simulink library "sm_excv_scene_lib"  (R2023a)
settings: Solver=VariableStepAuto  StartTime=0.0  StopTime=10.0  RelTol=1e-3
undefined symbols (not defined in the file): B1, B2, B3, B4, B5, B6, B7, B8, Excv, L1, L2, L3, L4, L5, L6, L7, L8, L9, Road, S1, S2, Scene, Scene_Data, SceneData, X, Y, Z
libraries: sm_lib x65, sm_tracked_vehicle_lib x47, $bdroot x45, nesl_utility x10
(part 2 of 3)

== system sm_excv_scene_lib/Grid Surface Terrain 1 Track ==
  CF Track Terrain L : sm_tracked_vehicle_lib/CF Track Terrain Full  K_Road=Scene.Contact.Terrain.K  B_Road=Scene.Contact.Terrain.B  TW_Road=Scene.Contact.Terrain.TW  F_dyn_Road=Scene.Contact.Terrain.mud  F_stat_Road=Scene.Contact.Terrain.mus  CV_Road=Scene.Contact.Terrain.CV
      settings: LibrarySourceBlock=sm_chain_drive_lib/CF_Road_Full
  Grid Surface : sm_lib/Curves and Surfaces/Grid Surface  XGridVector=Scene.Terrain.xg  XGridVectorUnits=m  YGridVector=Scene.Terrain.yg  YGridVectorUnits=m  ZHeights=Scene.Terrain.z_heights_data  ZHeightsUnits=m  GraphicType=FromGeometry  GraphicVisPropType=SimpleVisualProperties  GraphicDiffuseColor=[0.8196 0.7255 0.5098]  GraphicOpacity=1.0  GraphicSpecularColor=[0.5 0.5 0.5 1.0]  GraphicAmbientColor=[0.15 0.15 0.15 1.0]  GraphicEmissiveColor=[0.0 0.0 0.0 1.0]  GraphicShininess=75
  Transform Terrain : sm_lib/Frames and Transforms/Rigid Transform  TranslationMethod=Cartesian  TranslationStandardOffset=0  TranslationStandardOffsetUnits=m  TranslationStandardAxis=+Z  TranslationCartesianOffset="[-45 -45+2.5  -2.75+0.2]"  TranslationCartesianOffsetUnits=m  TranslationROffset=0  TranslationROffsetUnits=m  TranslationZOffset=0  TranslationZOffsetUnits=m  TranslationThetaOffset=0  TranslationThetaOffsetUnits=deg  RotationMethod=None  RotationAngleUnits=deg  RotationStandardAxis=+Z  RotationAngle=0.0  RotationArbitraryAxis=[0 0 1]  FollAlignAxisA=+X  BaseAlignAxisA=+Y  FollAlignAxisB=+Y  BaseAlignAxisB=+Z  RotationSequenceAxes=FollowerAxes  RotationSequence=XYX  RotationSequenceAngles=[0 0 0]  RotationSequenceAnglesUnits=deg  RotationMatrix=[1 0 0; 0 1 0; 0 0 1]  Quaternion=[1 0 0 0]
  W : PMIOPort  Side=Right
  L : PMIOPort  Port=2  Side=Left
  connections:
  CF Track Terrain L/RConn1 -- L/RConn1
  Transform Terrain/RConn1 -- Grid Surface/LConn1
  Grid Surface/RConn1 -- CF Track Terrain L/LConn1
  Transform Terrain/LConn1 -- W/RConn1

== system sm_excv_scene_lib/Grid Surface Terrain 2 Track ==
  CF Track Terrain L : sm_tracked_vehicle_lib/CF Track Terrain Full  K_Road=Scene.Contact.Terrain.K  B_Road=Scene.Contact.Terrain.B  TW_Road=Scene.Contact.Terrain.TW  F_dyn_Road=Scene.Contact.Terrain.mud  F_stat_Road=Scene.Contact.Terrain.mus  CV_Road=Scene.Contact.Terrain.CV
      settings: LibrarySourceBlock=sm_chain_drive_lib/CF_Road_Full
  CF Track Terrain R : sm_tracked_vehicle_lib/CF Track Terrain Full  K_Road=Scene.Contact.Terrain.K  B_Road=Scene.Contact.Terrain.B  TW_Road=Scene.Contact.Terrain.TW  F_dyn_Road=Scene.Contact.Terrain.mud  F_stat_Road=Scene.Contact.Terrain.mus  CV_Road=Scene.Contact.Terrain.CV
      settings: LibrarySourceBlock=sm_chain_drive_lib/CF_Road_Full
  Grid Surface : sm_lib/Curves and Surfaces/Grid Surface  XGridVector=Scene.Terrain.xg  XGridVectorUnits=m  YGridVector=Scene.Terrain.yg  YGridVectorUnits=m  ZHeights=Scene.Terrain.z_heights_data  ZHeightsUnits=m  GraphicType=FromGeometry  GraphicVisPropType=SimpleVisualProperties  GraphicDiffuseColor=[0.8196 0.7255 0.5098]  GraphicOpacity=1.0  GraphicSpecularColor=[0.5 0.5 0.5 1.0]  GraphicAmbientColor=[0.15 0.15 0.15 1.0]  GraphicEmissiveColor=[0.0 0.0 0.0 1.0]  GraphicShininess=75
  Transform Terrain : sm_lib/Frames and Transforms/Rigid Transform  TranslationMethod=Cartesian  TranslationStandardOffset=0  TranslationStandardOffsetUnits=m  TranslationStandardAxis=+Z  TranslationCartesianOffset="[-45 -45+2.5  -2.75+0.2]"  TranslationCartesianOffsetUnits=m  TranslationROffset=0  TranslationROffsetUnits=m  TranslationZOffset=0  TranslationZOffsetUnits=m  TranslationThetaOffset=0  TranslationThetaOffsetUnits=deg  RotationMethod=None  RotationAngleUnits=deg  RotationStandardAxis=+Z  RotationAngle=0.0  RotationArbitraryAxis=[0 0 1]  FollAlignAxisA=+X  BaseAlignAxisA=+Y  FollAlignAxisB=+Y  BaseAlignAxisB=+Z  RotationSequenceAxes=FollowerAxes  RotationSequence=XYX  RotationSequenceAngles=[0 0 0]  RotationSequenceAnglesUnits=deg  RotationMatrix=[1 0 0; 0 1 0; 0 0 1]  Quaternion=[1 0 0 0]
  W : PMIOPort  Side=Right
  L : PMIOPort  Port=2  Side=Left
  R : PMIOPort  Port=3  Side=Left
  connections:
  Transform Terrain/LConn1 -- W/RConn1
  CF Track Terrain R/LConn1 -- CF Track Terrain L/LConn1 -- Grid Surface/RConn1
  Transform Terrain/RConn1 -- Grid Surface/LConn1
  CF Track Terrain L/RConn1 -- L/RConn1
  R/RConn1 -- CF Track Terrain R/RConn1

== system sm_excv_scene_lib/Grid Surface Slope 1 Rollers ==
  CF Track Terrain L : sm_tracked_vehicle_lib/CF Roller Terrain Full  K_Road=K_Road  B_Road=B_Road  TW_Road=TW_Road  F_dyn_Road=F_dyn_Road  F_stat_Road=F_stat_Road  CV_Road=CV_Road
  Grid Surface Slope : $bdroot/Grid Surface Slope  road_len=road_len  road_wid=road_wid  slope_run=slope_run  slope_rise=slope_rise  slope_x0=slope_x0  slope_xres=slope_xres  surface_clr=surface_clr  surface_opc=surface_opc
  W : PMIOPort  Side=Right
  L : PMIOPort  Port=2  Side=Left
  connections:
  CF Track Terrain L/LConn1 -- Grid Surface Slope/LConn1
  Grid Surface Slope/RConn1 -- W/RConn1
  CF Track Terrain L/RConn1 -- L/RConn1

== system sm_excv_scene_lib/Grid Surface Slope 2 Rollers ==
  CF Track Terrain L : sm_tracked_vehicle_lib/CF Roller Terrain Full  K_Road=K_Road  B_Road=B_Road  TW_Road=TW_Road  F_dyn_Road=F_dyn_Road  F_stat_Road=F_stat_Road  CV_Road=CV_Road
  CF Track Terrain R : sm_tracked_vehicle_lib/CF Roller Terrain Full  K_Road=K_Road  B_Road=B_Road  TW_Road=TW_Road  F_dyn_Road=F_dyn_Road  F_stat_Road=F_stat_Road  CV_Road=CV_Road
  Grid Surface Slope : $bdroot/Grid Surface Slope  road_len=road_len  road_wid=road_wid  slope_run=slope_run  slope_rise=slope_rise  slope_x0=slope_x0  slope_xres=slope_xres  surface_clr=surface_clr  surface_opc=surface_opc
  W : PMIOPort  Side=Right
  L : PMIOPort  Port=2  Side=Left
  R : PMIOPort  Port=3  Side=Left
  connections:
  CF Track Terrain L/RConn1 -- L/RConn1
  Grid Surface Slope/RConn1 -- W/RConn1
  CF Track Terrain L/LConn1 -- CF Track Terrain R/LConn1 -- Grid Surface Slope/LConn1
  CF Track Terrain R/RConn1 -- R/RConn1

== system sm_excv_scene_lib/Grid Surface Terrain 1 Rollers ==
  CF Roller Terrain Full : sm_tracked_vehicle_lib/CF Roller Terrain Full  K_Road=Scene.Contact.Terrain.K  B_Road=Scene.Contact.Terrain.B  TW_Road=Scene.Contact.Terrain.TW  F_dyn_Road=Scene.Contact.Terrain.mud  F_stat_Road=Scene.Contact.Terrain.mus  CV_Road=Scene.Contact.Terrain.CV
  Grid Surface : sm_lib/Curves and Surfaces/Grid Surface  XGridVector=Scene.Terrain.xg  XGridVectorUnits=m  YGridVector=Scene.Terrain.yg  YGridVectorUnits=m  ZHeights=Scene.Terrain.z_heights_data  ZHeightsUnits=m  GraphicType=FromGeometry  GraphicVisPropType=SimpleVisualProperties  GraphicDiffuseColor=[0.8196 0.7255 0.5098]  GraphicOpacity=1.0  GraphicSpecularColor=[0.5 0.5 0.5 1.0]  GraphicAmbientColor=[0.15 0.15 0.15 1.0]  GraphicEmissiveColor=[0.0 0.0 0.0 1.0]  GraphicShininess=75
  Transform Terrain : sm_lib/Frames and Transforms/Rigid Transform  TranslationMethod=Cartesian  TranslationStandardOffset=0  TranslationStandardOffsetUnits=m  TranslationStandardAxis=+Z  TranslationCartesianOffset="[-45 -45+2.5  -2.75+0.2]"  TranslationCartesianOffsetUnits=m  TranslationROffset=0  TranslationROffsetUnits=m  TranslationZOffset=0  TranslationZOffsetUnits=m  TranslationThetaOffset=0  TranslationThetaOffsetUnits=deg  RotationMethod=None  RotationAngleUnits=deg  RotationStandardAxis=+Z  RotationAngle=0.0  RotationArbitraryAxis=[0 0 1]  FollAlignAxisA=+X  BaseAlignAxisA=+Y  FollAlignAxisB=+Y  BaseAlignAxisB=+Z  RotationSequenceAxes=FollowerAxes  RotationSequence=XYX  RotationSequenceAngles=[0 0 0]  RotationSequenceAnglesUnits=deg  RotationMatrix=[1 0 0; 0 1 0; 0 0 1]  Quaternion=[1 0 0 0]
  W : PMIOPort  Side=Right
  L : PMIOPort  Port=2  Side=Left
  connections:
  Transform Terrain/RConn1 -- Grid Surface/LConn1
  CF Roller Terrain Full/LConn1 -- Grid Surface/RConn1
  Transform Terrain/LConn1 -- W/RConn1
  CF Roller Terrain Full/RConn1 -- L/RConn1

== system sm_excv_scene_lib/Grid Surface Terrain 2 Rollers ==
  CF Roller Terrain L : sm_tracked_vehicle_lib/CF Roller Terrain Full  K_Road=Scene.Contact.Terrain.K  B_Road=Scene.Contact.Terrain.B  TW_Road=Scene.Contact.Terrain.TW  F_dyn_Road=Scene.Contact.Terrain.mud  F_stat_Road=Scene.Contact.Terrain.mus  CV_Road=Scene.Contact.Terrain.CV
  CF Roller Terrain R : sm_tracked_vehicle_lib/CF Roller Terrain Full  K_Road=Scene.Contact.Terrain.K  B_Road=Scene.Contact.Terrain.B  TW_Road=Scene.Contact.Terrain.TW  F_dyn_Road=Scene.Contact.Terrain.mud  F_stat_Road=Scene.Contact.Terrain.mus  CV_Road=Scene.Contact.Terrain.CV
  Grid Surface : sm_lib/Curves and Surfaces/Grid Surface  XGridVector=Scene.Terrain.xg  XGridVectorUnits=m  YGridVector=Scene.Terrain.yg  YGridVectorUnits=m  ZHeights=Scene.Terrain.z_heights_data  ZHeightsUnits=m  GraphicType=FromGeometry  GraphicVisPropType=SimpleVisualProperties  GraphicDiffuseColor=[0.8196 0.7255 0.5098]  GraphicOpacity=1.0  GraphicSpecularColor=[0.5 0.5 0.5 1.0]  GraphicAmbientColor=[0.15 0.15 0.15 1.0]  GraphicEmissiveColor=[0.0 0.0 0.0 1.0]  GraphicShininess=75
  Transform Terrain : sm_lib/Frames and Transforms/Rigid Transform  TranslationMethod=Cartesian  TranslationStandardOffset=0  TranslationStandardOffsetUnits=m  TranslationStandardAxis=+Z  TranslationCartesianOffset="[-45 -45+2.5  -2.75+0.2]"  TranslationCartesianOffsetUnits=m  TranslationROffset=0  TranslationROffsetUnits=m  TranslationZOffset=0  TranslationZOffsetUnits=m  TranslationThetaOffset=0  TranslationThetaOffsetUnits=deg  RotationMethod=None  RotationAngleUnits=deg  RotationStandardAxis=+Z  RotationAngle=0.0  RotationArbitraryAxis=[0 0 1]  FollAlignAxisA=+X  BaseAlignAxisA=+Y  FollAlignAxisB=+Y  BaseAlignAxisB=+Z  RotationSequenceAxes=FollowerAxes  RotationSequence=XYX  RotationSequenceAngles=[0 0 0]  RotationSequenceAnglesUnits=deg  RotationMatrix=[1 0 0; 0 1 0; 0 0 1]  Quaternion=[1 0 0 0]
  L : PMIOPort  Side=Left
  W : PMIOPort  Port=2  Side=Right
  R : PMIOPort  Port=3  Side=Left
  connections:
  CF Roller Terrain L/RConn1 -- L/RConn1
  Transform Terrain/LConn1 -- W/RConn1
  CF Roller Terrain L/LConn1 -- CF Roller Terrain R/LConn1 -- Grid Surface/RConn1
  Transform Terrain/RConn1 -- Grid Surface/LConn1
  R/RConn1 -- CF Roller Terrain R/RConn1

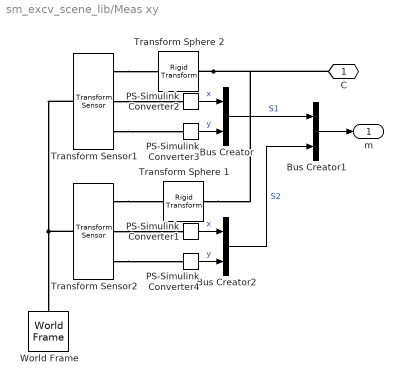
== system sm_excv_scene_lib/Meas xy ==
  Bus Creator : BusCreator  Inputs=2
  Bus Creator1 : BusCreator  Inputs=2
  Bus Creator2 : BusCreator  Inputs=2
  PS-Simulink Converter{1..4} (4 alike) : nesl_utility/PS-Simulink Converter  PhysicalDomain=network_engine_domain  SubClassName=ps_output  LeftPortType=input  RightPortType=output  PseudoPeriodic=off  Frequencies=[]  VectorFormat=inherit  Unit=inherit  AffineConversion=off
  Transform Sensor1 : sm_lib/Frames and Transforms/Transform Sensor  MeasurementFrame=World  RotationSequence=XYX  SenseAngle=off  SenseAxis=off  SenseQ=off  SenseR=off  SenseRotationSequence=off  SenseOmegaX=off  SenseOmegaY=off  SenseOmegaZ=off  SenseQDot=off  SenseRDot=off  SenseRotationSequenceDot=off  SenseAlphaX=off  SenseAlphaY=off  SenseAlphaZ=off  SenseQDDot=off  SenseRDDot=off  SenseX=on  SenseY=on  SenseZ=off  SenseRad=off  SenseAzim=off  SenseDist=off  SenseInc=off  SenseXDot=off  SenseYDot=off  SenseZDot=off  SenseRadDot=off  SenseAzimDot=off  SenseDistDot=off  SenseIncDot=off  SenseXDDot=off  SenseYDDot=off  SenseZDDot=off  SenseRadDDot=off  SenseAzimDDot=off  SenseDistDDot=off  SenseIncDDot=off
  Transform Sensor2 : sm_lib/Frames and Transforms/Transform Sensor  MeasurementFrame=World  RotationSequence=XYX  SenseAngle=off  SenseAxis=off  SenseQ=off  SenseR=off  SenseRotationSequence=off  SenseOmegaX=off  SenseOmegaY=off  SenseOmegaZ=off  SenseQDot=off  SenseRDot=off  SenseRotationSequenceDot=off  SenseAlphaX=off  SenseAlphaY=off  SenseAlphaZ=off  SenseQDDot=off  SenseRDDot=off  SenseX=on  SenseY=on  SenseZ=off  SenseRad=off  SenseAzim=off  SenseDist=off  SenseInc=off  SenseXDot=off  SenseYDot=off  SenseZDot=off  SenseRadDot=off  SenseAzimDot=off  SenseDistDot=off  SenseIncDot=off  SenseXDDot=off  SenseYDDot=off  SenseZDDot=off  SenseRadDDot=off  SenseAzimDDot=off  SenseDistDDot=off  SenseIncDDot=off
  Transform Sphere 1 : sm_lib/Frames and Transforms/Rigid Transform  TranslationMethod=StandardAxis  TranslationStandardOffset=whl_offset/2  TranslationStandardOffsetUnits=m  TranslationStandardAxis=+Z  TranslationCartesianOffset=[0 0 0]  TranslationCartesianOffsetUnits=m  TranslationROffset=0  TranslationROffsetUnits=m  TranslationZOffset=0  TranslationZOffsetUnits=m  TranslationThetaOffset=0  TranslationThetaOffsetUnits=deg  RotationMethod=None  RotationAngleUnits=deg  RotationStandardAxis=+Z  RotationAngle=0.0  RotationArbitraryAxis=[0 0 1]  FollAlignAxisA=+X  BaseAlignAxisA=+Y  FollAlignAxisB=+Y  BaseAlignAxisB=+Z  RotationSequenceAxes=FollowerAxes  RotationSequence=XYX  RotationSequenceAngles=[0 0 0]  RotationSequenceAnglesUnits=deg  RotationMatrix=[1 0 0; 0 1 0; 0 0 1]  Quaternion=[1 0 0 0]
  Transform Sphere 2 : sm_lib/Frames and Transforms/Rigid Transform  TranslationMethod=StandardAxis  TranslationStandardOffset=-whl_offset/2  TranslationStandardOffsetUnits=m  TranslationStandardAxis=+Z  TranslationCartesianOffset=[0 0 0]  TranslationCartesianOffsetUnits=m  TranslationROffset=0  TranslationROffsetUnits=m  TranslationZOffset=0  TranslationZOffsetUnits=m  TranslationThetaOffset=0  TranslationThetaOffsetUnits=deg  RotationMethod=None  RotationAngleUnits=deg  RotationStandardAxis=+Z  RotationAngle=0.0  RotationArbitraryAxis=[0 0 1]  FollAlignAxisA=+X  BaseAlignAxisA=+Y  FollAlignAxisB=+Y  BaseAlignAxisB=+Z  RotationSequenceAxes=FollowerAxes  RotationSequence=XYX  RotationSequenceAngles=[0 0 0]  RotationSequenceAnglesUnits=deg  RotationMatrix=[1 0 0; 0 1 0; 0 0 1]  Quaternion=[1 0 0 0]
  World Frame : sm_lib/Frames and Transforms/World Frame
  C : PMIOPort  Side=Left
  m : Outport
  wires:
  PS-Simulink Converter4/1 -> Bus Creator2/2  "y"
  PS-Simulink Converter1/1 -> Bus Creator2/1  "x"
  Bus Creator2/1 -> Bus Creator1/2  "S2"
  Bus Creator1/1 -> m/1
  Bus Creator/1 -> Bus Creator1/1  "S1"
  PS-Simulink Converter2/1 -> Bus Creator/1  "x"
  PS-Simulink Converter3/1 -> Bus Creator/2  "y"
  connections:
  Transform Sensor2/RConn1 -- Transform Sphere 1/RConn1
  Transform Sensor2/RConn3 -- PS-Simulink Converter4/LConn1
  Transform Sensor2/RConn2 -- PS-Simulink Converter1/LConn1
  Transform Sphere 2/LConn1 -- C/RConn1 -- Transform Sphere 1/LConn1
  Transform Sensor1/RConn2 -- PS-Simulink Converter2/LConn1
  Transform Sensor1/RConn1 -- Transform Sphere 2/RConn1
  Transform Sensor1/RConn3 -- PS-Simulink Converter3/LConn1
  Transform Sensor2/LConn1 -- Transform Sensor1/LConn1 -- World Frame/RConn1

== system sm_excv_scene_lib/Mesh ==
  Solid : sm_lib/Body Elements/Extruded Solid  GraphicAmbientColor=[0.15 0.15 0.15 1.0]  BasedOnType=Density  CenterOfMass=[0 0 0]  CenterOfMassUnits=m  GraphicDiffuseColor=mesh_color  ExportConvexHullGeometry=off  ExtrusionCrossSection=mesh_xsec  ExtrusionCrossSectionUnits=m  Density=mesh_rho  DensityUnits=kg/(m^3)  DoExposeReferenceFrame=on  GraphicEmissiveColor=[0.0 0.0 0.0 1.0]  ExportEntireGeometry=off  ExtrusionLength=mesh_thickness  ExtrusionLengthUnits=m  ExtrusionType=General  SerializedFrames=<Frames><Frame><Id>Frame1</Id><Value><Name>F</Name><Origin><Source>GeometricFeature</Source><FeatureName>top surface</FeatureName></Origin><PrimaryAxis><DefinedDirection>+Z</DefinedDirection><Source>ReferenceFrame</Source><SourceDirection>+Z</SourceDirection><FeatureName></FeatureName></PrimaryAxis><SecondaryAxis><DefinedDirection>+X</DefinedDirection><Source>ReferenceFrame</Source><SourceDirection>+X</SourceDirection><FeatureName></FeatureName></SecondaryAxis></Value></Frame><Frame><Id>Frame2</Id><Value><Name>B</Name><Origin><Source>GeometricFeature</Source><FeatureName>bottom surface</FeatureName></Origin><PrimaryAxis><DefinedDirection>+Z</DefinedDirection><Source>ReferenceFrame</Source><SourceDirection>+Z</SourceDirection><FeatureName></FeatureName></PrimaryAxis><SecondaryAxis><DefinedDirection>+X</DefinedDirection><Source>ReferenceFrame</Source><SourceDirection>+X</SourceDirection><FeatureName></FeatureName></SecondaryAxis></Value></Frame></Frames>  MarkerShape=Sphere  MarkerSize=10  GraphicType=FromGeometry  InertiaType=CalculateFromGeometry  Mass=1  MassUnits=kg  MomentsOfInertia=[1 1 1]  MomentsOfInertiaUnits=kg*m^2  PolygonNumSides=3  GraphicOpacity=mesh_opc  PolygonOuterRadius=1  PolygonOuterRadiusUnits=m  ProductsOfInertia=[0 0 0]  ProductsOfInertiaUnits=kg*m^2  GraphicShininess=75  GraphicSpecularColor=[0.5 0.5 0.5 1.0]  GraphicVisPropType=SimpleVisualProperties
  F : PMIOPort  Side=Right
  R : PMIOPort  Port=2  Side=Left
  B : PMIOPort  Port=3  Side=Right
  connections:
  B/RConn1 -- Solid/LConn2
  F/RConn1 -- Solid/LConn1
  Solid/RConn1 -- R/RConn1

== system sm_excv_scene_lib/Plateau 1 Roller Spheres ==
  mL : Inport
  Plateau : $bdroot/Road Profile and Grid  VariantControl=Plateau  RDF_Polyline=Scene.Plateau  grid_z_offset=0  grid_x=Scene.Grid.length*0.7  grid_y=Scene.Grid.width*0.01  grid_z=Scene.Grid.depth  grid_line_width=Scene.Grid.linewidth  grid_num_sq_x=Scene.Grid.numsquaresx*0.7  grid_num_sq_y=Scene.Grid.numsquaresy*0.01  plane_clr=Scene.Grid.planecolor  grid_clr=Scene.Grid.linecolor  grid_opc=1
      settings: LibrarySourceBlock=sm_excv_uneven_road_lib/Plateau
  Plateau L : $bdroot/Wheel Center to Patch 2x Roller Set  road_pz_x=Scene.Plateau.Road.pzLUT.px  road_pz_z=Scene.Plateau.Road.pzLUT.pz(:,1)  road_qy_x=Scene.Plateau.Road.qyLUT.px  road_qy_qy=Scene.Plateau.Road.qyLUT.qy(:,1)  tfilter=0.01  NormalStiffness=Scene.Contact.Terrain.K  NormalDamping=Scene.Contact.Terrain.B  NormalTransitionRegionWidth=Scene.Contact.Terrain.TW  CoefficientOfDynamicFriction=Scene.Contact.Terrain.mud  CoefficientOfStaticFriction=Scene.Contact.Terrain.mus  FrictionalCriticalVelocity=Scene.Contact.Terrain.CV  patch_x=Scene.Patch.w  patch_y=Scene.Patch.l  patch_clr=Scene.Patch.clr  patch_opc=Scene.Patch.opc
      settings: LibrarySourceBlock=sm_excv_uneven_road_lib/Rollers Rough Road1
  L : PMIOPort  Side=Right
  W : PMIOPort  Port=2  Side=Right
  wires:
  mL/1 -> Plateau L/1
  connections:
  Plateau L/RConn1 -- L/RConn1
  Plateau/RConn1 -- W/RConn1

== system sm_excv_scene_lib/Plateau 2 Rollers Spheres ==
  mL : Inport
  mR : Inport  Port=2
  Plateau : $bdroot/Road Profile and Grid  VariantControl=Plateau  RDF_Polyline=Scene.Plateau  grid_z_offset=0  grid_x=Scene.Grid.length*0.7  grid_y=Scene.Grid.width*0.01  grid_z=Scene.Grid.depth  grid_line_width=Scene.Grid.linewidth  grid_num_sq_x=Scene.Grid.numsquaresx*0.7  grid_num_sq_y=Scene.Grid.numsquaresy*0.01  plane_clr=Scene.Grid.planecolor  grid_clr=Scene.Grid.linecolor  grid_opc=1
      settings: LibrarySourceBlock=sm_excv_uneven_road_lib/Plateau
  Plateau L : $bdroot/Wheel Center to Patch 2x Roller Set  road_pz_x=Scene.Plateau.Road.pzLUT.px  road_pz_z=Scene.Plateau.Road.pzLUT.pz(:,1)  road_qy_x=Scene.Plateau.Road.qyLUT.px  road_qy_qy=Scene.Plateau.Road.qyLUT.qy(:,1)  tfilter=0.01  NormalStiffness=Scene.Contact.Terrain.K  NormalDamping=Scene.Contact.Terrain.B  NormalTransitionRegionWidth=Scene.Contact.Terrain.TW  CoefficientOfDynamicFriction=Scene.Contact.Terrain.mud  CoefficientOfStaticFriction=Scene.Contact.Terrain.mus  FrictionalCriticalVelocity=Scene.Contact.Terrain.CV  patch_x=Scene.Patch.w  patch_y=Scene.Patch.l  patch_clr=Scene.Patch.clr  patch_opc=Scene.Patch.opc
      settings: LibrarySourceBlock=sm_excv_uneven_road_lib/Rollers Rough Road1
  Plateau R : $bdroot/Wheel Center to Patch 2x Roller Set  road_pz_x=Scene.Plateau.Road.pzLUT.px  road_pz_z=Scene.Plateau.Road.pzLUT.pz(:,2)  road_qy_x=Scene.Plateau.Road.qyLUT.px  road_qy_qy=Scene.Plateau.Road.qyLUT.qy(:,2)  tfilter=0.01  NormalStiffness=Scene.Contact.Terrain.K  NormalDamping=Scene.Contact.Terrain.B  NormalTransitionRegionWidth=Scene.Contact.Terrain.TW  CoefficientOfDynamicFriction=Scene.Contact.Terrain.mud  CoefficientOfStaticFriction=Scene.Contact.Terrain.mus  FrictionalCriticalVelocity=Scene.Contact.Terrain.CV  patch_x=Scene.Patch.w  patch_y=Scene.Patch.l  patch_clr=Scene.Patch.clr  patch_opc=Scene.Patch.opc
      settings: LibrarySourceBlock=sm_excv_uneven_road_lib/Rollers Rough Road1
  L : PMIOPort  Side=Right
  W : PMIOPort  Port=2  Side=Right
  R : PMIOPort  Port=3  Side=Right
  wires:
  mL/1 -> Plateau L/1
  mR/1 -> Plateau R/1
  connections:
  Plateau R/RConn1 -- R/RConn1
  Plateau/RConn1 -- W/RConn1
  Plateau L/RConn1 -- L/RConn1

== system sm_excv_scene_lib/Road 1 Rollers ==
  CF Road Roller L : $bdroot/CF Road Rollers L  SystemSampleTime=-1  VariantActivationTime=update diagram  Latency=0  AutoFrameSizeCalculation=off
      settings: LibrarySourceBlock=|
      | sm_excv_scene_lib/CF
      | Road
      | Roller L
  Road Bumps : $bdroot/Road Bumps  road_x=Scene.Road.len  road_y=Scene.Road.wid  road_z=Scene.Road.hgt  bump_x=Scene.Road.Bump.len  bump_y=Scene.Road.Bump.wid  bump_z=Scene.Road.Bump.hgt  bloc_y=Scene.Road.Bump.offsety  bloc_z=Scene.Road.Bump.offsetz  bump_x0=Scene.Road.Bump.startx  bloc_dx=Scene.Road.Bump.deltax
  W : PMIOPort  Side=Right
  L : PMIOPort  Port=2  Side=Left
  connections:
  W/RConn1 -- Road Bumps/RConn1
  CF Road Roller L/LConn1 -- Road Bumps/LConn1
  CF Road Roller L/RConn1 -- L/RConn1

== system sm_excv_scene_lib/Road 1 Track ==
  CF Road Track L : $bdroot/CF Road Track L  SystemSampleTime=-1  VariantActivationTime=update diagram  Latency=0  AutoFrameSizeCalculation=off
  Road Bumps : $bdroot/Road Bumps  road_x=Scene.Road.len  road_y=Scene.Road.wid  road_z=Scene.Road.hgt  bump_x=Scene.Road.Bump.len  bump_y=Scene.Road.Bump.wid  bump_z=Scene.Road.Bump.hgt  bloc_y=Scene.Road.Bump.offsety  bloc_z=Scene.Road.Bump.offsetz  bump_x0=Scene.Road.Bump.startx  bloc_dx=Scene.Road.Bump.deltax
  W : PMIOPort  Side=Right
  L : PMIOPort  Port=2  Side=Left
  connections:
  CF Road Track L/RConn1 -- L/RConn1
  Road Bumps/LConn1 -- CF Road Track L/LConn1
  W/RConn1 -- Road Bumps/RConn1

== system sm_excv_scene_lib/Road 2 Rollers ==
  CF Road Roller L : $bdroot/CF Road Rollers L  SystemSampleTime=-1  VariantActivationTime=update diagram  Latency=0  AutoFrameSizeCalculation=off
      settings: LibrarySourceBlock=|
      | sm_excv_scene_lib/CF
      | Road
      | Roller L
  CF Road Rollers R : $bdroot/CF Road Rollers R  SystemSampleTime=-1  VariantActivationTime=update diagram  Latency=0  AutoFrameSizeCalculation=off
      settings: LibrarySourceBlock=|
      | sm_excv_scene_lib/CF
      | Road
      | Rollers R
  Road Bumps : $bdroot/Road Bumps  road_x=Scene.Road.len  road_y=Scene.Road.wid  road_z=Scene.Road.hgt  bump_x=Scene.Road.Bump.len  bump_y=Scene.Road.Bump.wid  bump_z=Scene.Road.Bump.hgt  bloc_y=Scene.Road.Bump.offsety  bloc_z=Scene.Road.Bump.offsetz  bump_x0=Scene.Road.Bump.startx  bloc_dx=Scene.Road.Bump.deltax
  W : PMIOPort  Side=Right
  L : PMIOPort  Port=2  Side=Left
  R : PMIOPort  Port=3  Side=Left
  connections:
  CF Road Roller L/RConn1 -- L/RConn1
  CF Road Roller L/LConn1 -- CF Road Rollers R/LConn1 -- Road Bumps/LConn1
  W/RConn1 -- Road Bumps/RConn1
  R/RConn1 -- CF Road Rollers R/RConn1

== system sm_excv_scene_lib/Road 2 Rollers Spheres ==
  CF Road Rollers Spheres L : $bdroot/CF Road Rollers Spheres L  SystemSampleTime=-1  VariantActivationTime=update diagram  Latency=0  AutoFrameSizeCalculation=off
  CF Road Rollers Spheres R : $bdroot/CF Road Rollers Spheres R  SystemSampleTime=-1  VariantActivationTime=update diagram  Latency=0  AutoFrameSizeCalculation=off
  Road Bumps : $bdroot/Road Bumps  road_x=Scene.Road.len  road_y=Scene.Road.wid  road_z=Scene.Road.hgt  bump_x=Scene.Road.Bump.len  bump_y=Scene.Road.Bump.wid  bump_z=Scene.Road.Bump.hgt  bloc_y=Scene.Road.Bump.offsety  bloc_z=Scene.Road.Bump.offsetz  bump_x0=Scene.Road.Bump.startx  bloc_dx=Scene.Road.Bump.deltax
  W : PMIOPort  Side=Right
  L : PMIOPort  Port=2  Side=Left
  R : PMIOPort  Port=3  Side=Left
  connections:
  CF Road Rollers Spheres R/RConn1 -- R/RConn1
  W/RConn1 -- Road Bumps/RConn1
  CF Road Rollers Spheres L/LConn1 -- CF Road Rollers Spheres R/LConn1 -- Road Bumps/LConn1
  CF Road Rollers Spheres L/RConn1 -- L/RConn1

== system sm_excv_scene_lib/Road 2 Track ==
  CF Road Track L : $bdroot/CF Road Track L  SystemSampleTime=-1  VariantActivationTime=update diagram  Latency=0  AutoFrameSizeCalculation=off
  CF Road Track R : $bdroot/CF Road Track R  SystemSampleTime=-1  VariantActivationTime=update diagram  Latency=0  AutoFrameSizeCalculation=off
  Road Bumps : $bdroot/Road Bumps  road_x=Scene.Road.len  road_y=Scene.Road.wid  road_z=Scene.Road.hgt  bump_x=Scene.Road.Bump.len  bump_y=Scene.Road.Bump.wid  bump_z=Scene.Road.Bump.hgt  bloc_y=Scene.Road.Bump.offsety  bloc_z=Scene.Road.Bump.offsetz  bump_x0=Scene.Road.Bump.startx  bloc_dx=Scene.Road.Bump.deltax
  W : PMIOPort  Side=Right
  L : PMIOPort  Port=2  Side=Left
  R : PMIOPort  Port=3  Side=Left
  connections:
  CF Road Track L/LConn1 -- Road Bumps/LConn1 -- CF Road Track R/LConn1
  CF Road Track L/RConn1 -- L/RConn1
  CF Road Track R/RConn1 -- R/RConn1
  W/RConn1 -- Road Bumps/RConn1

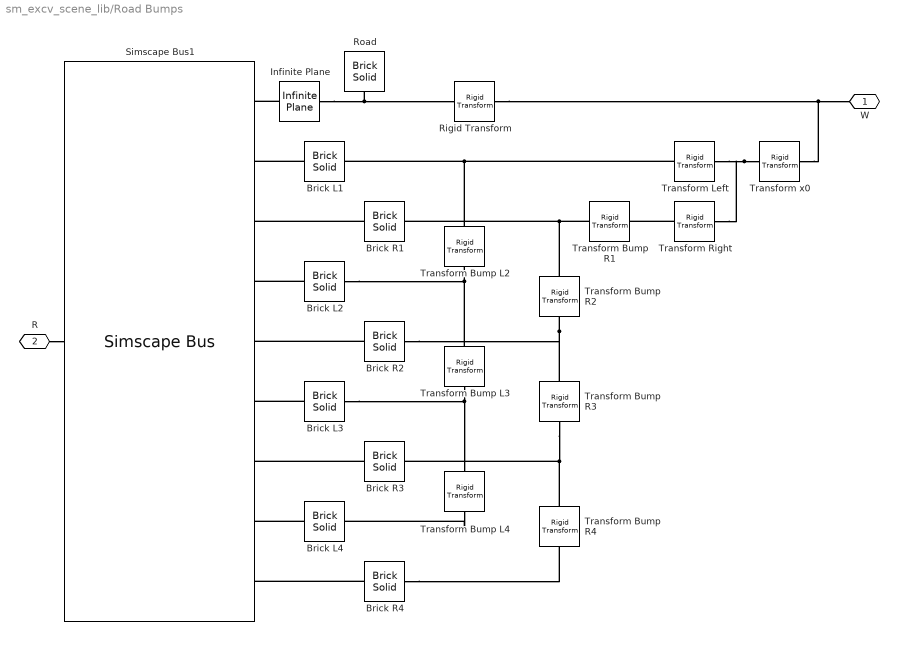
== system sm_excv_scene_lib/Road Bumps ==
  Brick L{1..4} (4 alike) : sm_lib/Body Elements/Brick Solid  GraphicAmbientColor=[0.15 0.15 0.15 1.0]  BasedOnType=Density  BrickDimensions=[bump_x bump_y bump_z]  BrickDimensionsUnits=m  CenterOfMass=[0 0 0]  CenterOfMassUnits=m  GraphicDiffuseColor=[0.6 0.6 0.0]  Density=1000  DensityUnits=kg/m^3  DoExposeReferenceFrame=off  GraphicEmissiveColor=[0.0 0.0 0.0 1.0]  ExportEntireGeometry=on  SerializedFrames=<Frames><Frame><Id>Frame1</Id><Value><Name>F1</Name><Origin><Source>GeometricFeature</Source><FeatureName>-z surface</FeatureName></Origin><PrimaryAxis><DefinedDirection>+Z</DefinedDirection><Source>ReferenceFrame</Source><SourceDirection>+Z</SourceDirection><FeatureName></FeatureName></PrimaryAxis><SecondaryAxis><DefinedDirection>+X</DefinedDirection><Source>ReferenceFrame</Source><SourceDirection>+X</SourceDirection><FeatureName></FeatureName></SecondaryAxis></Value></Frame></Frames>  MarkerShape=Sphere  MarkerSize=10  GraphicType=FromGeometry  InertiaType=CalculateFromGeometry  Mass=1  MassUnits=kg  MomentsOfInertia=[1 1 1]  MomentsOfInertiaUnits=kg*m^2  GraphicOpacity=1.0  ProductsOfInertia=[0 0 0]  ProductsOfInertiaUnits=kg*m^2  GraphicShininess=75  GraphicSpecularColor=[0.5 0.5 0.5 1.0]  GraphicVisPropType=SimpleVisualProperties
  Brick R{1..4} (4 alike) : sm_lib/Body Elements/Brick Solid  GraphicAmbientColor=[0.15 0.15 0.15 1.0]  BasedOnType=Density  BrickDimensions=[bump_x bump_y bump_z]  BrickDimensionsUnits=m  CenterOfMass=[0 0 0]  CenterOfMassUnits=m  GraphicDiffuseColor=[0.6 0.6 0.0]  Density=1000  DensityUnits=kg/m^3  DoExposeReferenceFrame=off  GraphicEmissiveColor=[0.0 0.0 0.0 1.0]  ExportEntireGeometry=on  SerializedFrames=<Frames><Frame><Id>Frame1</Id><Value><Name>F1</Name><Origin><Source>GeometricFeature</Source><FeatureName>-z surface</FeatureName></Origin><PrimaryAxis><DefinedDirection>+Z</DefinedDirection><Source>ReferenceFrame</Source><SourceDirection>+Z</SourceDirection><FeatureName></FeatureName></PrimaryAxis><SecondaryAxis><DefinedDirection>+X</DefinedDirection><Source>ReferenceFrame</Source><SourceDirection>+X</SourceDirection><FeatureName></FeatureName></SecondaryAxis></Value></Frame></Frames>  MarkerShape=Sphere  MarkerSize=10  GraphicType=FromGeometry  InertiaType=CalculateFromGeometry  Mass=1  MassUnits=kg  MomentsOfInertia=[1 1 1]  MomentsOfInertiaUnits=kg*m^2  GraphicOpacity=1.0  ProductsOfInertia=[0 0 0]  ProductsOfInertiaUnits=kg*m^2  GraphicShininess=75  GraphicSpecularColor=[0.5 0.5 0.5 1.0]  GraphicVisPropType=SimpleVisualProperties
  Infinite Plane : sm_lib/Curves and Surfaces/Infinite Plane  GraphicType=None  GraphicPlaneWidth=50  GraphicPlaneWidthUnits=m  GraphicPlaneHeight=50  GraphicPlaneHeightUnits=m  GraphicVisPropType=SimpleVisualProperties  GraphicDiffuseColor=[0.5 0.5 0.5]  GraphicOpacity=0.25  GraphicSpecularColor=[0.5 0.5 0.5 1.0]  GraphicAmbientColor=[0.15 0.15 0.15 1.0]  GraphicEmissiveColor=[0.0 0.0 0.0 1.0]  GraphicShininess=75
  Rigid Transform : sm_lib/Frames and Transforms/Rigid Transform  TranslationMethod=Cartesian  TranslationStandardOffset=0  TranslationStandardOffsetUnits=m  TranslationStandardAxis=+Z  TranslationCartesianOffset=[road_x/2-0.5 0 0]  TranslationCartesianOffsetUnits=m  TranslationROffset=0  TranslationROffsetUnits=m  TranslationZOffset=0  TranslationZOffsetUnits=m  TranslationThetaOffset=0  TranslationThetaOffsetUnits=deg  RotationMethod=None  RotationAngleUnits=deg  RotationStandardAxis=+Z  RotationAngle=0.0  RotationArbitraryAxis=[0 0 1]  FollAlignAxisA=+X  BaseAlignAxisA=+Y  FollAlignAxisB=+Y  BaseAlignAxisB=+Z  RotationSequenceAxes=FollowerAxes  RotationSequence=XYX  RotationSequenceAngles=[0 0 0]  RotationSequenceAnglesUnits=deg  RotationMatrix=[1 0 0; 0 1 0; 0 0 1]  Quaternion=[1 0 0 0]
  Road : sm_lib/Body Elements/Brick Solid  GraphicAmbientColor=[0.15 0.15 0.15 1.0]  BasedOnType=Density  BrickDimensions=[road_x road_y road_z]  BrickDimensionsUnits=m  CenterOfMass=[0 0 0]  CenterOfMassUnits=m  GraphicDiffuseColor=[0.43529412 0.3372549 0.3372549]  Density=1000  DensityUnits=kg/m^3  DoExposeReferenceFrame=off  GraphicEmissiveColor=[0.0 0.0 0.0 1.0]  ExportEntireGeometry=off  SerializedFrames=<Frames><Frame><Id>Frame1</Id><Value><Name>F1</Name><Origin><Source>GeometricFeature</Source><FeatureName>+z surface</FeatureName></Origin><PrimaryAxis><DefinedDirection>+Z</DefinedDirection><Source>ReferenceFrame</Source><SourceDirection>+Z</SourceDirection><FeatureName></FeatureName></PrimaryAxis><SecondaryAxis><DefinedDirection>+X</DefinedDirection><Source>ReferenceFrame</Source><SourceDirection>+X</SourceDirection><FeatureName></FeatureName></SecondaryAxis></Value></Frame></Frames>  MarkerShape=Sphere  MarkerSize=10  GraphicType=FromGeometry  InertiaType=CalculateFromGeometry  Mass=1  MassUnits=kg  MomentsOfInertia=[1 1 1]  MomentsOfInertiaUnits=kg*m^2  GraphicOpacity=0.2  ProductsOfInertia=[0 0 0]  ProductsOfInertiaUnits=kg*m^2  GraphicShininess=75  GraphicSpecularColor=[0.5 0.5 0.5 1.0]  GraphicVisPropType=SimpleVisualProperties
  Simscape Bus1 : SimscapeBus  HierarchyStrings=Road;B1;B2;B3;B4;B5;B6;B7;B8  ConnectionType=Bus: Road_CBO
  Transform Bump L2 : sm_lib/Frames and Transforms/Rigid Transform  TranslationMethod=StandardAxis  TranslationStandardOffset=bloc_dx*2  TranslationStandardOffsetUnits=m  TranslationStandardAxis=+X  TranslationCartesianOffset=[0 0 0]  TranslationCartesianOffsetUnits=m  TranslationROffset=0  TranslationROffsetUnits=m  TranslationZOffset=0  TranslationZOffsetUnits=m  TranslationThetaOffset=0  TranslationThetaOffsetUnits=deg  RotationMethod=None  RotationAngleUnits=deg  RotationStandardAxis=+Z  RotationAngle=0.0  RotationArbitraryAxis=[0 0 1]  FollAlignAxisA=+X  BaseAlignAxisA=+Y  FollAlignAxisB=+Y  BaseAlignAxisB=+Z  RotationSequenceAxes=FollowerAxes  RotationSequence=XYX  RotationSequenceAngles=[0 0 0]  RotationSequenceAnglesUnits=deg  RotationMatrix=[1 0 0; 0 1 0; 0 0 1]  Quaternion=[1 0 0 0]
  Transform Bump L3 : sm_lib/Frames and Transforms/Rigid Transform  TranslationMethod=StandardAxis  TranslationStandardOffset=bloc_dx*2  TranslationStandardOffsetUnits=m  TranslationStandardAxis=+X  TranslationCartesianOffset=[0 0 0]  TranslationCartesianOffsetUnits=m  TranslationROffset=0  TranslationROffsetUnits=m  TranslationZOffset=0  TranslationZOffsetUnits=m  TranslationThetaOffset=0  TranslationThetaOffsetUnits=deg  RotationMethod=None  RotationAngleUnits=deg  RotationStandardAxis=+Z  RotationAngle=0.0  RotationArbitraryAxis=[0 0 1]  FollAlignAxisA=+X  BaseAlignAxisA=+Y  FollAlignAxisB=+Y  BaseAlignAxisB=+Z  RotationSequenceAxes=FollowerAxes  RotationSequence=XYX  RotationSequenceAngles=[0 0 0]  RotationSequenceAnglesUnits=deg  RotationMatrix=[1 0 0; 0 1 0; 0 0 1]  Quaternion=[1 0 0 0]
  Transform Bump L4 : sm_lib/Frames and Transforms/Rigid Transform  TranslationMethod=StandardAxis  TranslationStandardOffset=bloc_dx*2  TranslationStandardOffsetUnits=m  TranslationStandardAxis=+X  TranslationCartesianOffset=[0 0 0]  TranslationCartesianOffsetUnits=m  TranslationROffset=0  TranslationROffsetUnits=m  TranslationZOffset=0  TranslationZOffsetUnits=m  TranslationThetaOffset=0  TranslationThetaOffsetUnits=deg  RotationMethod=None  RotationAngleUnits=deg  RotationStandardAxis=+Z  RotationAngle=0.0  RotationArbitraryAxis=[0 0 1]  FollAlignAxisA=+X  BaseAlignAxisA=+Y  FollAlignAxisB=+Y  BaseAlignAxisB=+Z  RotationSequenceAxes=FollowerAxes  RotationSequence=XYX  RotationSequenceAngles=[0 0 0]  RotationSequenceAnglesUnits=deg  RotationMatrix=[1 0 0; 0 1 0; 0 0 1]  Quaternion=[1 0 0 0]
  Transform Bump R1 : sm_lib/Frames and Transforms/Rigid Transform  TranslationMethod=StandardAxis  TranslationStandardOffset=bloc_dx  TranslationStandardOffsetUnits=m  TranslationStandardAxis=+X  TranslationCartesianOffset=[0 0 0]  TranslationCartesianOffsetUnits=m  TranslationROffset=0  TranslationROffsetUnits=m  TranslationZOffset=0  TranslationZOffsetUnits=m  TranslationThetaOffset=0  TranslationThetaOffsetUnits=deg  RotationMethod=None  RotationAngleUnits=deg  RotationStandardAxis=+Z  RotationAngle=0.0  RotationArbitraryAxis=[0 0 1]  FollAlignAxisA=+X  BaseAlignAxisA=+Y  FollAlignAxisB=+Y  BaseAlignAxisB=+Z  RotationSequenceAxes=FollowerAxes  RotationSequence=XYX  RotationSequenceAngles=[0 0 0]  RotationSequenceAnglesUnits=deg  RotationMatrix=[1 0 0; 0 1 0; 0 0 1]  Quaternion=[1 0 0 0]
  Transform Bump R2 : sm_lib/Frames and Transforms/Rigid Transform  TranslationMethod=StandardAxis  TranslationStandardOffset=bloc_dx*2  TranslationStandardOffsetUnits=m  TranslationStandardAxis=+X  TranslationCartesianOffset=[0 0 0]  TranslationCartesianOffsetUnits=m  TranslationROffset=0  TranslationROffsetUnits=m  TranslationZOffset=0  TranslationZOffsetUnits=m  TranslationThetaOffset=0  TranslationThetaOffsetUnits=deg  RotationMethod=None  RotationAngleUnits=deg  RotationStandardAxis=+Z  RotationAngle=0.0  RotationArbitraryAxis=[0 0 1]  FollAlignAxisA=+X  BaseAlignAxisA=+Y  FollAlignAxisB=+Y  BaseAlignAxisB=+Z  RotationSequenceAxes=FollowerAxes  RotationSequence=XYX  RotationSequenceAngles=[0 0 0]  RotationSequenceAnglesUnits=deg  RotationMatrix=[1 0 0; 0 1 0; 0 0 1]  Quaternion=[1 0 0 0]
  Transform Bump R3 : sm_lib/Frames and Transforms/Rigid Transform  TranslationMethod=StandardAxis  TranslationStandardOffset=bloc_dx*2  TranslationStandardOffsetUnits=m  TranslationStandardAxis=+X  TranslationCartesianOffset=[0 0 0]  TranslationCartesianOffsetUnits=m  TranslationROffset=0  TranslationROffsetUnits=m  TranslationZOffset=0  TranslationZOffsetUnits=m  TranslationThetaOffset=0  TranslationThetaOffsetUnits=deg  RotationMethod=None  RotationAngleUnits=deg  RotationStandardAxis=+Z  RotationAngle=0.0  RotationArbitraryAxis=[0 0 1]  FollAlignAxisA=+X  BaseAlignAxisA=+Y  FollAlignAxisB=+Y  BaseAlignAxisB=+Z  RotationSequenceAxes=FollowerAxes  RotationSequence=XYX  RotationSequenceAngles=[0 0 0]  RotationSequenceAnglesUnits=deg  RotationMatrix=[1 0 0; 0 1 0; 0 0 1]  Quaternion=[1 0 0 0]
  Transform Bump R4 : sm_lib/Frames and Transforms/Rigid Transform  TranslationMethod=StandardAxis  TranslationStandardOffset=bloc_dx*2  TranslationStandardOffsetUnits=m  TranslationStandardAxis=+X  TranslationCartesianOffset=[0 0 0]  TranslationCartesianOffsetUnits=m  TranslationROffset=0  TranslationROffsetUnits=m  TranslationZOffset=0  TranslationZOffsetUnits=m  TranslationThetaOffset=0  TranslationThetaOffsetUnits=deg  RotationMethod=None  RotationAngleUnits=deg  RotationStandardAxis=+Z  RotationAngle=0.0  RotationArbitraryAxis=[0 0 1]  FollAlignAxisA=+X  BaseAlignAxisA=+Y  FollAlignAxisB=+Y  BaseAlignAxisB=+Z  RotationSequenceAxes=FollowerAxes  RotationSequence=XYX  RotationSequenceAngles=[0 0 0]  RotationSequenceAnglesUnits=deg  RotationMatrix=[1 0 0; 0 1 0; 0 0 1]  Quaternion=[1 0 0 0]
  Transform Left : sm_lib/Frames and Transforms/Rigid Transform  TranslationMethod=StandardAxis  TranslationStandardOffset=bloc_y  TranslationStandardOffsetUnits=m  TranslationStandardAxis=+Y  TranslationCartesianOffset=[0 0 0]  TranslationCartesianOffsetUnits=m  TranslationROffset=0  TranslationROffsetUnits=m  TranslationZOffset=0  TranslationZOffsetUnits=m  TranslationThetaOffset=0  TranslationThetaOffsetUnits=deg  RotationMethod=None  RotationAngleUnits=deg  RotationStandardAxis=+Z  RotationAngle=0.0  RotationArbitraryAxis=[0 0 1]  FollAlignAxisA=+X  BaseAlignAxisA=+Y  FollAlignAxisB=+Y  BaseAlignAxisB=+Z  RotationSequenceAxes=FollowerAxes  RotationSequence=XYX  RotationSequenceAngles=[0 0 0]  RotationSequenceAnglesUnits=deg  RotationMatrix=[1 0 0; 0 1 0; 0 0 1]  Quaternion=[1 0 0 0]
  Transform Right : sm_lib/Frames and Transforms/Rigid Transform  TranslationMethod=StandardAxis  TranslationStandardOffset=bloc_y  TranslationStandardOffsetUnits=m  TranslationStandardAxis=-Y  TranslationCartesianOffset=[0 0 0]  TranslationCartesianOffsetUnits=m  TranslationROffset=0  TranslationROffsetUnits=m  TranslationZOffset=0  TranslationZOffsetUnits=m  TranslationThetaOffset=0  TranslationThetaOffsetUnits=deg  RotationMethod=None  RotationAngleUnits=deg  RotationStandardAxis=+Z  RotationAngle=0.0  RotationArbitraryAxis=[0 0 1]  FollAlignAxisA=+X  BaseAlignAxisA=+Y  FollAlignAxisB=+Y  BaseAlignAxisB=+Z  RotationSequenceAxes=FollowerAxes  RotationSequence=XYX  RotationSequenceAngles=[0 0 0]  RotationSequenceAnglesUnits=deg  RotationMatrix=[1 0 0; 0 1 0; 0 0 1]  Quaternion=[1 0 0 0]
  Transform x0 : sm_lib/Frames and Transforms/Rigid Transform  TranslationMethod=StandardAxis  TranslationStandardOffset=bump_x0  TranslationStandardOffsetUnits=m  TranslationStandardAxis=+X  TranslationCartesianOffset=[0 0 0]  TranslationCartesianOffsetUnits=m  TranslationROffset=0  TranslationROffsetUnits=m  TranslationZOffset=0  TranslationZOffsetUnits=m  TranslationThetaOffset=0  TranslationThetaOffsetUnits=deg  RotationMethod=None  RotationAngleUnits=deg  RotationStandardAxis=+X  RotationAngle=0.0  RotationArbitraryAxis=[0 0 1]  FollAlignAxisA=+X  BaseAlignAxisA=+Y  FollAlignAxisB=+Y  BaseAlignAxisB=+Z  RotationSequenceAxes=FollowerAxes  RotationSequence=XYX  RotationSequenceAngles=[0 0 0]  RotationSequenceAnglesUnits=deg  RotationMatrix=[1 0 0; 0 1 0; 0 0 1]  Quaternion=[1 0 0 0]
  W : PMIOPort  Side=Right
  R : PMIOPort  Port=2  Side=Left
  connections:
  Infinite Plane/RConn1 -- Simscape Bus1/LConn1
  Transform Bump L2/LConn1 -- Brick L1/LConn1 -- Transform Left/RConn1
  Brick L1/RConn1 -- Simscape Bus1/LConn2
  Transform Bump R2/LConn1 -- Brick R1/LConn1 -- Transform Bump R1/RConn1
  Transform Bump R2/RConn1 -- Brick R2/LConn1 -- Transform Bump R3/LConn1
  Transform Bump L3/RConn1 -- Brick L3/LConn1 -- Transform Bump L4/LConn1
  Transform Bump R3/RConn1 -- Brick R3/LConn1 -- Transform Bump R4/LConn1
  Transform Bump L4/RConn1 -- Brick L4/LConn1
  Brick R4/LConn1 -- Transform Bump R4/RConn1
  Brick R1/RConn1 -- Simscape Bus1/LConn3
  Brick L2/RConn1 -- Simscape Bus1/LConn4
  Brick R2/RConn1 -- Simscape Bus1/LConn5
  Brick L3/RConn1 -- Simscape Bus1/LConn6
  Brick R3/RConn1 -- Simscape Bus1/LConn7
  Brick L4/RConn1 -- Simscape Bus1/LConn8
  Brick R4/RConn1 -- Simscape Bus1/LConn9
  Infinite Plane/LConn1 -- Rigid Transform/RConn1 -- Road/LConn1
  R/RConn1 -- Simscape Bus1/RConn1
  Transform x0/LConn1 -- Rigid Transform/LConn1 -- W/RConn1
  Transform x0/RConn1 -- Transform Left/LConn1 -- Transform Right/LConn1
  Brick L2/LConn1 -- Transform Bump L2/RConn1 -- Transform Bump L3/LConn1
  Transform Right/RConn1 -- Transform Bump R1/LConn1
